simulink model "sim_2_2"  (R2021b)
settings: Solver=ode4  StartTime=0.0  StopTime=tstop  FixedStep=tstep  RelTol=1e-3
values from neighbouring files (symbols this model uses):
  zeta = 0.1    [sim_2_part2.m]
undefined symbols (not defined in the file or in its folder): om_n
settings Model: Creator=shash  LastModifiedBy=shash
settings DataIOCC: ReturnWorkspaceOutputs=off

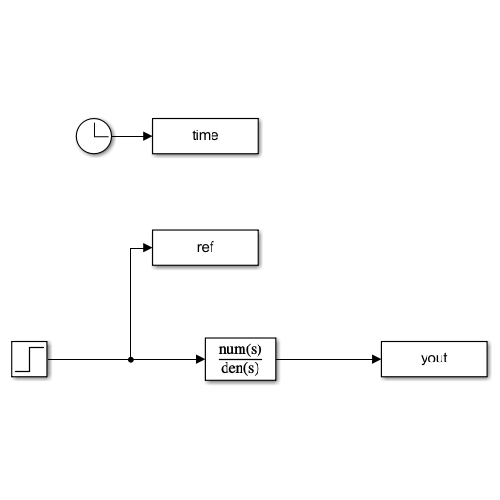
[thumbnail: Simulink's stored preview of the top-level diagram]
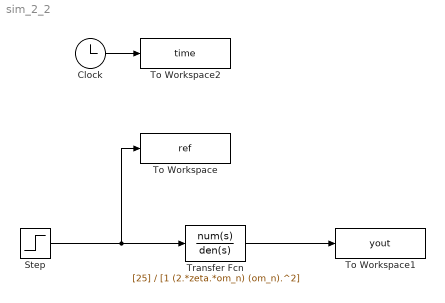
== system sim_2_2 ==
  Clock : Clock
  Step : Step  Time=0  SampleTime=0
  To Workspace : ToWorkspace  VariableName=ref  SampleTime=-1
  To Workspace1 : ToWorkspace  VariableName=yout  SampleTime=-1
  To Workspace2 : ToWorkspace  VariableName=time  SampleTime=-1
  Transfer Fcn : TransferFcn  Numerator=[25]  Denominator=[1 (2.*zeta.*om_n) (om_n).^2]
  wires:
  Step/1 -> To Workspace/1, Transfer Fcn/1
  Transfer Fcn/1 -> To Workspace1/1
  Clock/1 -> To Workspace2/1
